simulink model "getAngleBias"  (R2022a)
settings: Solver=ode5  StartTime=0.0  StopTime=30.0  RelTol=1e-3
undefined symbols (not defined in the file or in its folder): opts, Standard_Devices, Ts_udp, UDP_Protocol
libraries: dspstat3 x2, sharedtransform x1, sldrtlib x1
settings Model: Creator=Simonas  LastModifiedBy=Simonas
settings HardwareCC: ProdBitPerLong=64  ProdHWDeviceType=Intel->x86-64 (Linux 64)
settings RTWCC: Description=Simulink Desktop Real-Time  SystemTargetFile=sldrt.tlc  TemplateMakefile=sldrt.tmf  RTWCompilerOptimization=on
settings CodeAppCC: MaxIdLength=95
settings SimulinkDesktopRealTimeCC: TargetLibSuffix=_sldrt.a  TargetPreCompLibLocation=C:\Program Files\MATLAB\R2022a\toolbox\sldrt\lib\win64

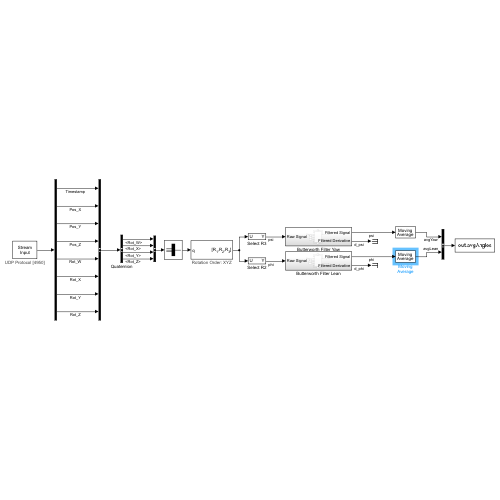
[thumbnail: Simulink's stored preview of the top-level diagram]
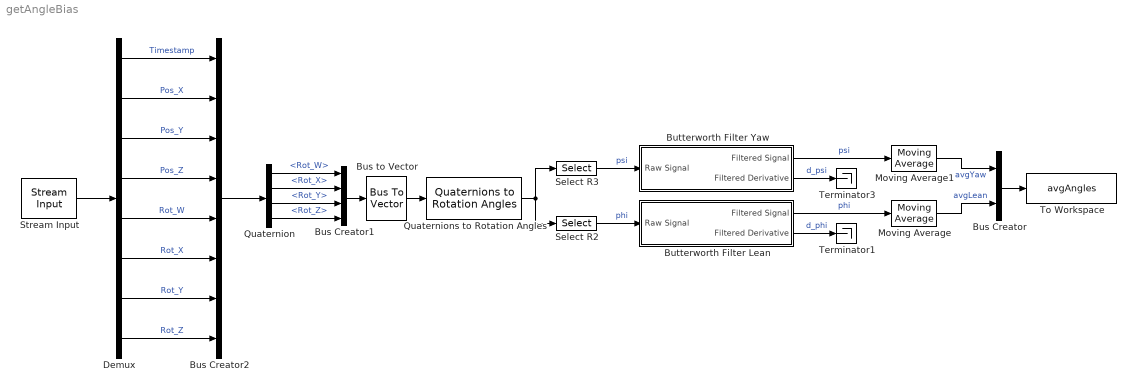
== system getAngleBias ==
  Bus Creator : BusCreator  Inputs=2
  Bus Creator1 : BusCreator  Inputs=4
  Bus Creator2 : BusCreator  Inputs=8
  Bus to Vector : BusToVector
  Butterworth Filter Lean : Subsystem
  Butterworth Filter Yaw : Subsystem
  Demux : Demux  Outputs=8
  Moving Average : dspstat3/Moving Average  Method=Sliding window  ForgettingFactorPort=off  SpecifyWindowLength=off  WindowLength=5/Ts_udp  ForgettingFactor=0.9  SimulateUsing=Code generation
  Moving Average1 : dspstat3/Moving Average  Method=Sliding window  ForgettingFactorPort=off  SpecifyWindowLength=off  WindowLength=5/Ts_udp  ForgettingFactor=0.9  SimulateUsing=Code generation
  Quaternion : BusSelector  OutputSignals=Rot_W,Rot_X,Rot_Y,Rot_Z
  Quaternions to Rotation Angles : sharedtransform/Quaternions to Rotation Angles  rotationOrder=XYZ  aMode=aMode
      settings: SourceProductBaseCode=AE,PW,DR,MT,VE
  Select R2 : Selector  InputPortWidth=3  IndexOptions=Index vector (dialog)  Indices=2  OutputSizes=1
  Select R3 : Selector  InputPortWidth=3  IndexOptions=Index vector (dialog)  Indices=3  OutputSizes=1
  Stream Input : sldrtlib/Stream Input  SampleTime=opts.T_udp  MaxMissedTicks=1000000  ShowMissedTicks=off  YieldWhenWaiting=on  DrvName=Standard_Devices/UDP_Protocol  DrvAddress=4950  DrvOptions=[0 16385 0 0 0 0 0 0 0 0 0 0 0 0 0 0 0 0 0 0 0 0 0 0 0 0 0 0 0 0 0 0 0 0 0 0 0 0 0 0 0 0 0 0 0 0 0 0 0 0 0 0 0 0 0 0 0 0 0 0 0 0 0 0 0 0 0 0 0 0 0 0 0 0 0 0 0 0 0 0 0 0 0 0 0 0 0 0 0 0 0 0 0 0 0 0 0 0 0 0 0 0 0 0 0 0 0 0 0 0 0 0 0 0 0 0 0 0 0 0 0 0 0 0 0 0 0 0 0 0 0 0 0 0 0 0 0 0 0 0 0 0 0 0 0 0 0 0 0 0 0 0 0 0 0 0 0 0 0 0 0 0 0 0 0 0 0 0 0 0 0 0 0 0 0 0 0 0 0 0 0 0 0 0 0 0 0 0 0 0 0 0 0 0 0 0 0 0 0 0 0 0 0 0 0 0 0 0 0 0 0 0 0 0 0 0 0 0 0 0 0 0 0 0 0 0 0 0 0 0 0 0 0 0 0 0 0 0 0 0 0 0 0 0 0 0 0 0 0 0 0 0 0 0 0 0]  DataTypes={'8*double'}  FormatString='%f,%f,%f,%f,%f,%f,%f,%f'  Terminator='\n'  ShowReady=off  ShowError=off
      settings: AttributesFormatString=UDP Protocol [4950]  SourceProductBaseCode=WT
  Terminator1 : Terminator
  Terminator3 : Terminator
  To Workspace : ToWorkspace  VariableName=avgAngles  SampleTime=-1
  wires:
  Demux/6 -> Bus Creator2/6  "Rot_X"
  Demux/2 -> Bus Creator2/2  "Pos_X"
  Demux/3 -> Bus Creator2/3  "Pos_Y"
  Demux/4 -> Bus Creator2/4  "Pos_Z"
  Demux/1 -> Bus Creator2/1  "Timestamp"
  Stream Input/1 -> Demux/1
  Demux/8 -> Bus Creator2/8  "Rot_Z"
  Demux/7 -> Bus Creator2/7  "Rot_Y"
  Demux/5 -> Bus Creator2/5  "Rot_W"
  Bus Creator/1 -> To Workspace/1
  Butterworth Filter Lean/2(Filtered Derivative) -> Terminator1/1  "d_phi"
  Moving Average1/1 -> Bus Creator/1  "avgYaw"
  Moving Average/1 -> Bus Creator/2  "avgLean"
  Butterworth Filter Yaw/2(Filtered Derivative) -> Terminator3/1  "d_psi"
  Butterworth Filter Yaw/1(Filtered Signal) -> Moving Average1/1  "psi"
  Select R3/1 -> Butterworth Filter Yaw/1(Raw Signal)  "psi"
  Butterworth Filter Lean/1(Filtered Signal) -> Moving Average/1  "phi"
  Quaternions to Rotation Angles/1 -> Select R3/1, Select R2/1
  Bus to Vector/1 -> Quaternions to Rotation Angles/1
  Bus Creator1/1 -> Bus to Vector/1
  Quaternion/1 -> Bus Creator1/1  "<Rot_W>"
  Select R2/1 -> Butterworth Filter Lean/1(Raw Signal)  "phi"
  Quaternion/4 -> Bus Creator1/4  "<Rot_Z>"
  Quaternion/3 -> Bus Creator1/3  "<Rot_Y>"
  Quaternion/2 -> Bus Creator1/2  "<Rot_X>"
  Bus Creator2/1 -> Quaternion/1

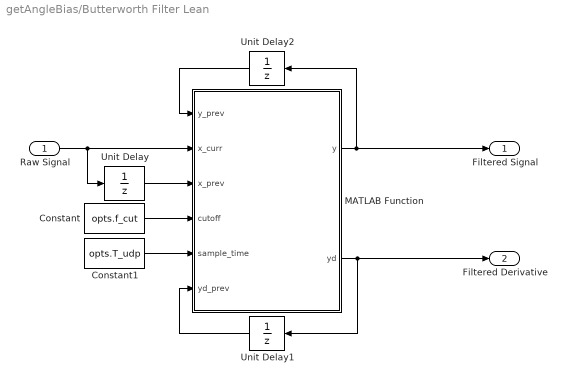
== system getAngleBias/Butterworth Filter Lean ==
  Raw Signal : Inport
  Constant : Constant  Value=opts.f_cut  SampleTime=opts.T_udp
  Constant1 : Constant  Value=opts.T_udp  SampleTime=opts.T_udp
  MATLAB Function : MATLAB Function  TreatAsAtomicUnit=on
  Unit Delay : UnitDelay  SampleTime=opts.T_udp  HasFrameUpgradeWarning=on
  Unit Delay1 : UnitDelay  SampleTime=opts.T_udp  HasFrameUpgradeWarning=on
  Unit Delay2 : UnitDelay  SampleTime=opts.T_udp  HasFrameUpgradeWarning=on
  Filtered Signal : Outport
  Filtered Derivative : Outport  Port=2
  wires:
  MATLAB Function/1(y) -> Unit Delay2/1, Filtered Signal/1
  MATLAB Function/2(yd) -> Unit Delay1/1, Filtered Derivative/1
  Raw Signal/1 -> Unit Delay/1, MATLAB Function/2(x_curr)
  Unit Delay/1 -> MATLAB Function/3(x_prev)
  Constant/1 -> MATLAB Function/4(cutoff)
  Constant1/1 -> MATLAB Function/5(sample_time)
  Unit Delay2/1 -> MATLAB Function/1(y_prev)
  Unit Delay1/1 -> MATLAB Function/6(yd_prev)

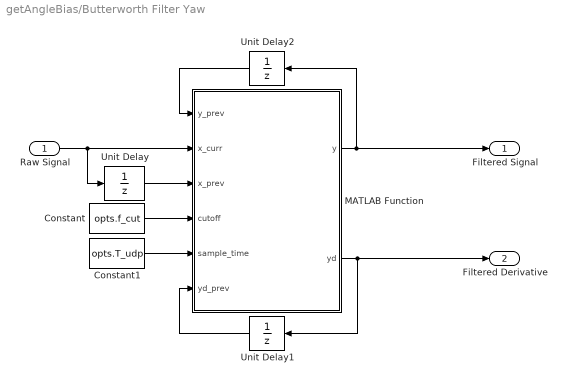
== system getAngleBias/Butterworth Filter Yaw ==
  Raw Signal : Inport
  Constant : Constant  Value=opts.f_cut  SampleTime=opts.T_udp
  Constant1 : Constant  Value=opts.T_udp  SampleTime=opts.T_udp
  MATLAB Function : MATLAB Function  TreatAsAtomicUnit=on
  Unit Delay : UnitDelay  SampleTime=opts.T_udp  HasFrameUpgradeWarning=on
  Unit Delay1 : UnitDelay  SampleTime=opts.T_udp  HasFrameUpgradeWarning=on
  Unit Delay2 : UnitDelay  SampleTime=opts.T_udp  HasFrameUpgradeWarning=on
  Filtered Signal : Outport
  Filtered Derivative : Outport  Port=2
  wires:
  MATLAB Function/1(y) -> Unit Delay2/1, Filtered Signal/1
  MATLAB Function/2(yd) -> Unit Delay1/1, Filtered Derivative/1
  Raw Signal/1 -> Unit Delay/1, MATLAB Function/2(x_curr)
  Unit Delay/1 -> MATLAB Function/3(x_prev)
  Constant/1 -> MATLAB Function/4(cutoff)
  Constant1/1 -> MATLAB Function/5(sample_time)
  Unit Delay2/1 -> MATLAB Function/1(y_prev)
  Unit Delay1/1 -> MATLAB Function/6(yd_prev)

== matlab function getAngleBias/Butterworth Filter Lean/MATLAB Function ==
  data: y_prev input; y output; x_curr input; x_prev input; cutoff input; sample_time input; yd_prev input; yd output
function [y, yd] = realtime_filter(y_prev, x_curr, x_prev, ...
                                   cutoff, sample_time, yd_prev)
a = (2*pi * cutoff^2);
b = sqrt(2) * 2*pi * cutoff;
h = sample_time;
denom = 4 + 2*h*b + h^2*a;

A = (4 + 2*h*b - h^2*a) / denom;
B = 4*h / denom;
C = -4*h*a / denom;
D = (4 - 2*h*b - h^2*a) / denom;
E = 2*h^2*a / denom;
F = 4*h*a / denom;

y = A * y_prev + B * yd_prev + E * (x_curr + x_prev) / 2;
yd = C * y_prev + D * yd_prev + F * (x_curr + x_prev) / 2;

== matlab function getAngleBias/Butterworth Filter Yaw/MATLAB Function ==
  data: y_prev input; y output; x_curr input; x_prev input; cutoff input; sample_time input; yd_prev input; yd output
function [y, yd] = realtime_filter(y_prev, x_curr, x_prev, ...
                                   cutoff, sample_time, yd_prev)
a = (2*pi * cutoff^2);
b = sqrt(2) * 2*pi * cutoff;
h = sample_time;
denom = 4 + 2*h*b + h^2*a;

A = (4 + 2*h*b - h^2*a) / denom;
B = 4*h / denom;
C = -4*h*a / denom;
D = (4 - 2*h*b - h^2*a) / denom;
E = 2*h^2*a / denom;
F = 4*h*a / denom;

y = A * y_prev + B * yd_prev + E * (x_curr + x_prev) / 2;
yd = C * y_prev + D * yd_prev + F * (x_curr + x_prev) / 2;
